simulink model "NCGPC_circulaire"  (R2016b)
settings: Solver=ode5  StartTime=0.0  StopTime=40  FixedStep=0.005  RelTol=1e-2
libraries: simulink x1
settings Model: Creator=amar  LastModifiedBy=fnadi

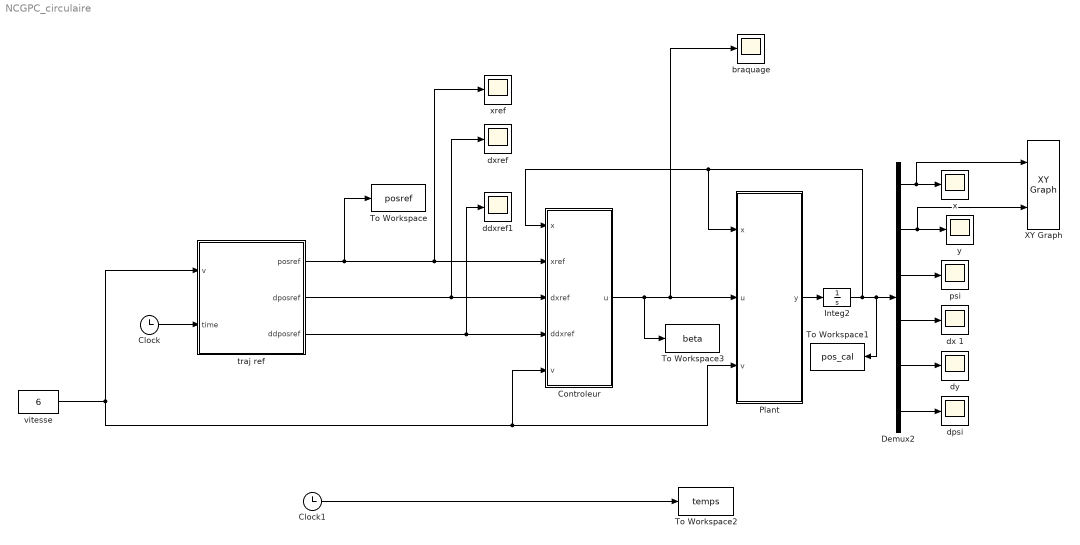
== system NCGPC_circulaire ==
  Clock : Clock
  Clock1 : Clock
  Controleur : MATLAB Function  TreatAsAtomicUnit=on
  Demux2 : Demux  Outputs=6
  Integ2 : Integrator  InitialCondition=[-60 0 -0.8*pi/2 0 -6 6/60]
  Plant : MATLAB Function  TreatAsAtomicUnit=on
  To Workspace : ToWorkspace  VariableName=posref  SampleTime=-1
  To Workspace1 : ToWorkspace  VariableName=pos_cal  SampleTime=-1
  To Workspace2 : ToWorkspace  VariableName=temps  SampleTime=-1
  To Workspace3 : ToWorkspace  VariableName=beta  SampleTime=-1
  XY Graph : simulink/Sinks/XY Graph  xmin=-50  xmax=50  ymin=-50  ymax=50  st=-1
  braquage : Scope
  ddxref1 : Scope
  dpsi : Scope
  dx 1 : Scope
  dxref : Scope
  dy : Scope
  psi : Scope
  traj ref : MATLAB Function  TreatAsAtomicUnit=on
  vitesse : Constant  Value=6
  "x " : Scope
  xref : Scope
  "y " : Scope
  wires:
  Plant/1(y) -> Integ2/1
  Demux2/5 -> dy/1
  Demux2/6 -> dpsi/1
  Demux2/4 -> dx 1/1
  Demux2/3 -> psi/1
  Demux2/2 -> XY Graph/2, "y "/1
  Demux2/1 -> XY Graph/1, "x "/1
  Integ2/1 -> Controleur/1(x), Plant/1(x), To Workspace1/1, Demux2/1
  vitesse/1 -> traj ref/1(v), Controleur/5(v), Plant/3(v)
  Clock/1 -> traj ref/2(time)
  Controleur/1(u) -> To Workspace3/1, Plant/2(u), braquage/1
  traj ref/3(ddposref) -> Controleur/4(ddxref), ddxref1/1
  traj ref/2(dposref) -> Controleur/3(dxref), dxref/1
  traj ref/1(posref) -> To Workspace/1, xref/1, Controleur/2(xref)
  Clock1/1 -> To Workspace2/1

== matlab function NCGPC_circulaire/Controleur ==
  data: x input; xref input; u output; dxref input; ddxref input; v input
function u = MPC(x,xref,dxref,ddxref,v)

%rigidité de dérive
Cf=10000;
Cr=10000;

%position du cdg
a=1.2;
b=1.2;

%masse et momet d'inertie
masse=700;
moment=400*(1.2^2+0.7^2)/12;

%vitesse
vit=v;

% temps de prédiction
Ts=6;

%%
psi=x(3);
Vpsi=x(6);
Vx=x(4)*cos(psi)+x(5)*sin(psi);
Vy=-x(4)*sin(psi)+x(5)*cos(psi);


%% matrice A et B
a11=2*(Cf+Cr)/(masse*vit);
a12=-2*(a*Cf-b*Cr)/(masse*vit)-vit;
a21=-2*(a*Cf-b*Cr)/(vit*moment);
a22=2*(a^2*Cf+b^2*Cr)/(vit*moment);

b11=2*Cf/masse; b12=-2*Cr/masse;
b21=-2*a*Cf/moment; b22=-2*b*Cr/moment;


%%
zetah=Vx*Vpsi+a11*Vy+a12*Vpsi;

%%

Ep=[x(1)-xref(1);
    x(4)-dxref(1);
    -zetah*sin(psi)-Vy*Vpsi*cos(psi)-ddxref(1);
    x(2)-xref(2);
    x(5)-dxref(2);
    zetah*cos(psi)-Vy*Vpsi*sin(psi)-ddxref(2);
    x(3)-xref(3);
    Vpsi-dxref(3);
    a21*Vy+a22*Vpsi-ddxref(3)];

D=[-b11*sin(psi) -b12*sin(psi);
   b11*cos(psi) b12*cos(psi);
   b21 b22];

Ki=[10/(3*Ts^2) 10/(4*Ts) 1];
ZE=zeros(1,3);

K= [Ki ZE ZE;
    ZE Ki ZE;
    ZE ZE Ki];

u=-inv(D'*D)*D'*K*Ep;

%u=[-0.2 0];

== matlab function NCGPC_circulaire/Plant ==
  data: x input; u input; v input; y output
function y = plant(x,u,v)

%global param

%rigidité de dérive
Cf=10000;
Cr=10000;

%position du cdg
a=1.2;
b=1.2;

%masse et momet d'inertie
masse=700;
moment=400*(1.2^2+0.7^2)/12;

%vitesse
vit=v;

%%
beta_f=u(1);
beta_r=u(2);

Xpos=x(1);
Ypos=x(2);
psi=x(3);

dXpos=x(4);
dYpos=x(5);
dpsi=x(6);

%% matrice A et B
a11=2*(Cf+Cr)/(masse*vit);
a12=-2*(a*Cf-b*Cr)/(masse*vit)-vit;
a21=-2*(a*Cf-b*Cr)/(vit*moment);
a22=2*(a^2*Cf+b^2*Cr)/(vit*moment);

b11=2*Cf/masse; b12=-2*Cr/masse;
b21=-2*a*Cf/moment; b22=-2*b*Cr/moment;

%%

R=[cos(psi) -sin(psi); sin(psi) cos(psi)];

V = R'*[dXpos; dYpos];
Vx=V(1);
Vy=V(2);

%%

dVx =0 ;
dVy = a11*Vy + a12*dpsi + b11*beta_f + b12*beta_r;
ddpsi = a21*Vy + a22*dpsi + b21*beta_f + b22*beta_r;

%%

acc = R*[dVx; dVy] + dpsi*[-Vx*sin(psi)-Vy*cos(psi); Vx*cos(psi)-Vy*sin(psi)] ;

ddXpos=acc(1); 
ddYpos=acc(2);

y = [x(4) x(5) x(6) ddXpos ddYpos ddpsi] ;

== matlab function NCGPC_circulaire/traj ref ==
  data: v input; time input; posref output; dposref output; ddposref output
function [posref,dposref,ddposref] = ref(v,time)

% %droite
% Xposref=v*time;
% Yposref=0;

%cercle
R=60;
T=2*pi*R/v;
omega=v/R;

teta=omega*time;


% psiref=pi/2+teta;
% Xposref=R*cos(teta);
% Yposref=R*sin(teta);
% 
% dpsiref=omega;
% dXposref=-R*omega*sin(teta);
% dYposref=R*omega*cos(teta);
% 
% ddpsiref=0;
% ddXposref=-R*omega^2*cos(teta);
% ddYposref=-R*omega^2*sin(teta);
% 
% posref=[Xposref Yposref psiref]; 
% dposref=[dXposref dYposref dpsiref];
% ddposref =[ddXposref ddYposref ddpsiref];
psiref=pi/2+teta-pi;
Xposref=R*sin(psiref);
Yposref=-R*cos(psiref);

dpsiref=omega;
dXposref=v*cos(psiref);
dYposref=v*sin(psiref);

ddpsiref=0;
ddXposref=-v^2/R*sin(psiref);
ddYposref=v^2/R*cos(psiref);

posref=[Xposref Yposref psiref]; 
dposref=[dXposref dYposref dpsiref];
ddposref =[ddXposref ddYposref ddpsiref];
